simulink model "aerodynamic_test"  (R2018a)
settings: Solver=VariableStepAuto  StartTime=0.0  StopTime=10.0  RelTol=1e-3
undefined symbols (not defined in the file or in its folder): Earth, WGS84
libraries: aerolibasang x2, aerolib6dof2 x1, aerolibadyn x1, aerolibatmos2 x1
settings Model: Creator=annakooperberg  LastModifiedBy=annakooperberg

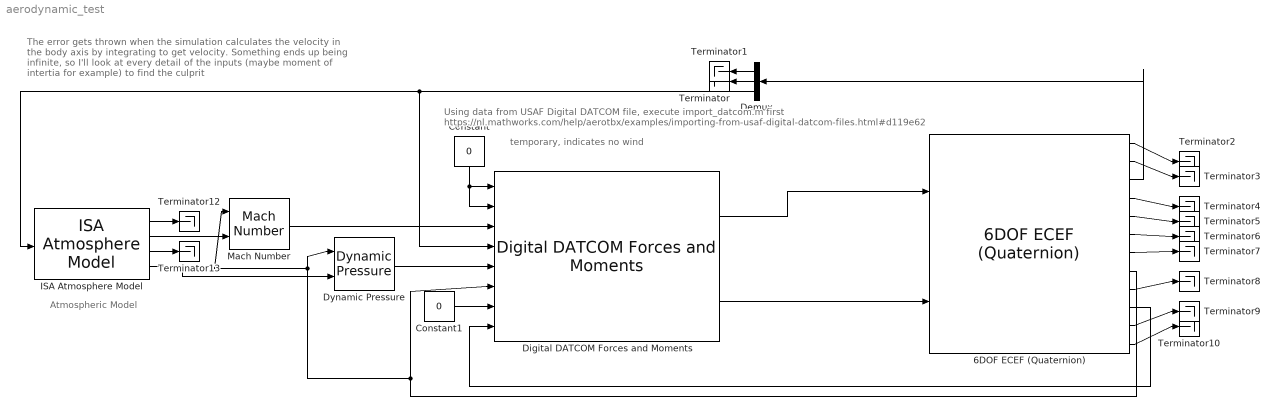
== system aerodynamic_test ==
  note: The error gets thrown when the simulation calculates the velocity in the body axis by integrating to get velocity. Something ends up being infinite, so I'll look at every detail of the inputs (maybe moment of intertia for example) to find the culprit
  note: Atmospheric Model
  note: Using data from USAF Digital DATCOM file, execute import_datcom.m first
      | https://nl.mathworks.com/help/aerotbx/examples/importing-from-usaf-digital-datcom-files.html#d119e62
  note: temporary,
      | indicates no
      | wind
  6DOF ECEF (Quaternion) : aerolib6dof2/6DOF ECEF (Quaternion)  units=Metric (MKS)  mtype=Fixed  xg_0=[0 0 0]  Vm_0=[0 0 0]  eul_0=[0 3*pi/8 0]  pm_0=[0 0 0]  mass_0=100  mass_e=0.5  mass_f=2.0  inertia=eye(3)  inertia_e=eye(3)  inertia_f=2*eye(3)  vre_flag=on  abi_flag=off  ptype=Earth (WGS84)  R=6378137  F=1/298.257223563  w_E=7292115e-11  angle_in=Internal  LG0=0
      settings: SourceProductName=Aerospace Blockset  SourceProductBaseCode=AE
  Constant : Constant  Value=0
  Constant1 : Constant  Value=0
  Demux : Demux  Outputs=3
  Digital DATCOM Forces and Moments : aerolibadyn/Digital DATCOM Forces and Moments  units=Metric (MKS)  dcase=data  fmode=Body  buildno=0  imethod=None - flat  emethod=None - clip  rmethod=Clip to Range  action=None
      settings: SourceProductName=Aerospace Blockset  SourceProductBaseCode=AE
  Dynamic Pressure : aerolibasang/Dynamic Pressure
  ISA Atmosphere Model : aerolibatmos2/ISA Atmosphere Model  custom=off  g=9.80665  gamma=1.4  R=287.0531  L=0.0065  h_trop=11000  h_strat=20000  rho0=1.225  P0=101325  T0=288.15  h0=0
      settings: SourceProductName=Aerospace Blockset
  Mach Number : aerolibasang/Mach Number
      settings: SourceProductName=Aerospace Blockset  SourceProductBaseCode=AE
  Terminator{,1..10,12..13} (13 alike) : Terminator
  wires:
  ISA Atmosphere Model/1 -> Terminator12/1
  ISA Atmosphere Model/3 -> Terminator13/1
  Digital DATCOM Forces and Moments/1 -> 6DOF ECEF (Quaternion)/1
  6DOF ECEF (Quaternion)/8 -> Digital DATCOM Forces and Moments/6, Dynamic Pressure/1, Mach Number/1
  ISA Atmosphere Model/2 -> Mach Number/2
  Digital DATCOM Forces and Moments/2 -> 6DOF ECEF (Quaternion)/2
  Mach Number/1 -> Digital DATCOM Forces and Moments/3
  Constant1/1 -> Digital DATCOM Forces and Moments/7
  ISA Atmosphere Model/4 -> Dynamic Pressure/2
  Dynamic Pressure/1 -> Digital DATCOM Forces and Moments/5
  Demux/3 -> ISA Atmosphere Model/1, Digital DATCOM Forces and Moments/4
  6DOF ECEF (Quaternion)/10 -> Digital DATCOM Forces and Moments/8
  Constant/1 -> Digital DATCOM Forces and Moments/2, Digital DATCOM Forces and Moments/1
  6DOF ECEF (Quaternion)/3 -> Demux/1
  Demux/2 -> Terminator/1
  Demux/1 -> Terminator1/1
  6DOF ECEF (Quaternion)/1 -> Terminator2/1
  6DOF ECEF (Quaternion)/2 -> Terminator3/1
  6DOF ECEF (Quaternion)/4 -> Terminator4/1
  6DOF ECEF (Quaternion)/5 -> Terminator5/1
  6DOF ECEF (Quaternion)/6 -> Terminator6/1
  6DOF ECEF (Quaternion)/7 -> Terminator7/1
  6DOF ECEF (Quaternion)/9 -> Terminator8/1
  6DOF ECEF (Quaternion)/11 -> Terminator9/1
  6DOF ECEF (Quaternion)/12 -> Terminator10/1
